simulink model "BO_NonLinear"  (R2024b)
settings: Solver=VariableStepAuto  StartTime=0.0  StopTime=10.0  RelTol=1e-3
values from neighbouring files (symbols this model uses):
  g = 9.81    [exo.m]    (also in parameters.m = 9.82; test_anime.m = params.g)
  k1 = 0.01    [parameters.m]
  k2 = 0.01    [parameters.m]
  l = params.l    [animate_pendulum_cart.m]    (also in animate_pendulum_cart_wheel_.m = params.L; exo.m = 1; parameters.m = 1)
  M = 1.5    [parameters.m]
  m = 0.5    [parameters.m]
settings Model: Creator=dsagn  LastModifiedBy=dsagn

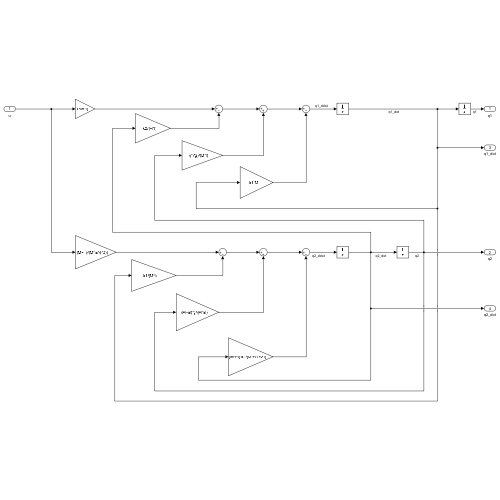
[thumbnail: Simulink's stored preview of the top-level diagram]
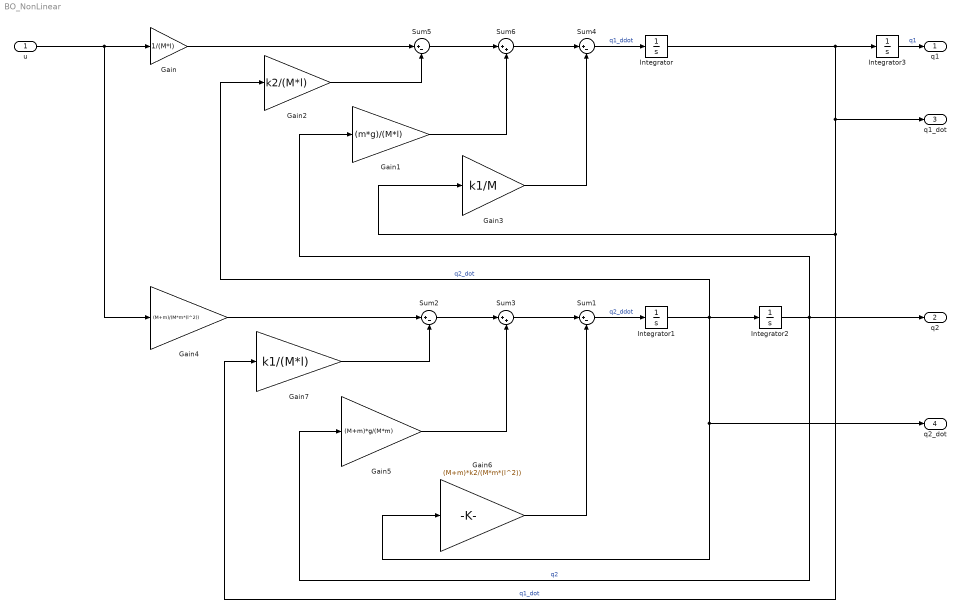
== system BO_NonLinear ==
  "u " : Inport
  Gain : Gain  Gain=1/(M*l)
  Gain1 : Gain  Gain=(m*g)/(M*l)
  Gain2 : Gain  Gain=k2/(M*l)
  Gain3 : Gain  Gain=k1/M
  Gain4 : Gain  Gain=(M+m)/(M*m*(l^2))
  Gain5 : Gain  Gain=(M+m)*g/(M*m)
  Gain6 : Gain  Gain=(M+m)*k2/(M*m*(l^2))
  Gain7 : Gain  Gain=k1/(M*l)
  Integrator : Integrator
  Integrator1 : Integrator
  Integrator2 : Integrator  InitialCondition=-90
  Integrator3 : Integrator
  Sum{1..2,4..5} (4 alike) : Sum  Inputs=|+-
  Sum3 : Sum  Inputs=|++
  Sum6 : Sum  Inputs=|++
  q1 : Outport  VectorParamsAs1DForOutWhenUnconnected=off
  "q2 " : Outport  Port=2  VectorParamsAs1DForOutWhenUnconnected=off
  q1_dot : Outport  Port=3  VectorParamsAs1DForOutWhenUnconnected=off
  q2_dot : Outport  Port=4  VectorParamsAs1DForOutWhenUnconnected=off
  wires:
  Gain7/1 -> Sum2/2
  Integrator2/1 -> "q2 "/1, Gain5/1, Gain1/1  "q2"
  Gain6/1 -> Sum1/2
  Sum1/1 -> Integrator1/1  "q2_ddot"
  Gain5/1 -> Sum3/2
  Gain1/1 -> Sum6/2
  Integrator1/1 -> q2_dot/1, Gain6/1, Gain2/1, Integrator2/1  "q2_dot"
  Sum5/1 -> Sum6/1
  Gain2/1 -> Sum5/2
  Integrator3/1 -> q1/1  "q1"
  Gain3/1 -> Sum4/2
  Sum3/1 -> Sum1/1
  Gain/1 -> Sum5/1
  Sum4/1 -> Integrator/1  "q1_ddot"
  Integrator/1 -> Integrator3/1, q1_dot/1, Gain7/1, Gain3/1  "q1_dot"
  Gain4/1 -> Sum2/1
  Sum6/1 -> Sum4/1
  "u "/1 -> Gain4/1, Gain/1
  Sum2/1 -> Sum3/1
